simulink model "local_maxima_findpeaks"  (R2019b)
settings: Solver=VariableStepAuto  StartTime=0.0  StopTime=10  RelTol=1e-3
libraries: simulink x2, hdlsllib x1
settings Model: Creator=sbuccelli  LastModifiedBy=sbuccelli

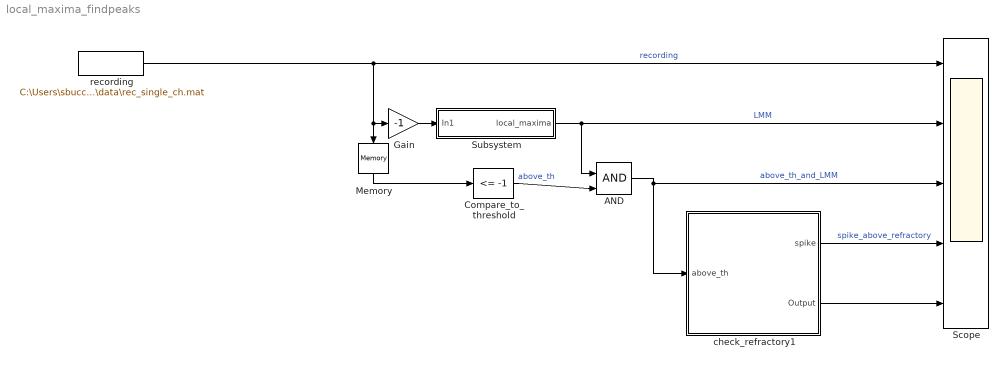
== system local_maxima_findpeaks ==
  AND : Logic  IconShape=distinctive  AllPortsSameDT=off  OutDataTypeStr=boolean
  Compare_to_threshold : simulink/Logic and Bit Operations/Compare To Constant  relop=<=  const=-1  OutDataTypeStr=boolean
  Gain : Gain  Gain=-1
  Memory : Memory  InheritSampleTime=on
  Scope : Scope  NumInputPorts=5
  Subsystem : Subsystem
  check_refractory1 : Subsystem
  recording : FromFile  FileName=C:\Users\sbuccelli\Documents\GitHub\closed-loop-neuroscience\data\rec_single_ch.mat  SampleTime=1/32e3
  wires:
  recording/1 -> Memory/1, Gain/1, Scope/1  "recording"
  AND/1 -> check_refractory1/1(above_th), Scope/3  "above_th_and_LMM"
  check_refractory1/1(spike) -> Scope/4  "spike_above_refractory"
  check_refractory1/2(Output) -> Scope/5
  Subsystem/1(local_maxima) -> AND/1, Scope/2  "LMM"
  Memory/1 -> Compare_to_threshold/1
  Compare_to_threshold/1 -> AND/2  "above_th"
  Gain/1 -> Subsystem/1(In1)

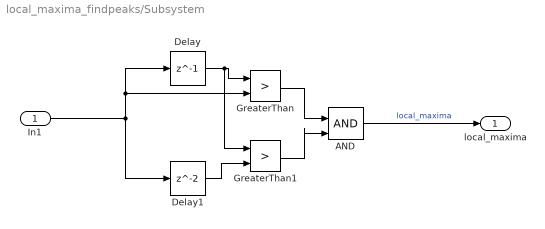
== system local_maxima_findpeaks/Subsystem ==
  In1 : Inport
  AND : Logic  IconShape=distinctive  AllPortsSameDT=off  OutDataTypeStr=boolean
  Delay : Delay  DelayLength=1
  Delay1 : Delay
  GreaterThan : RelationalOperator  Operator=>  OutDataTypeStr=boolean  RndMeth=Simplest
  GreaterThan1 : RelationalOperator  Operator=>  OutDataTypeStr=boolean  RndMeth=Simplest
  local_maxima : Outport
  wires:
  Delay1/1 -> GreaterThan1/2
  GreaterThan1/1 -> AND/2
  GreaterThan/1 -> AND/1
  Delay/1 -> GreaterThan1/1, GreaterThan/1
  AND/1 -> local_maxima/1  "local_maxima"
  In1/1 -> Delay/1, GreaterThan/2, Delay1/1

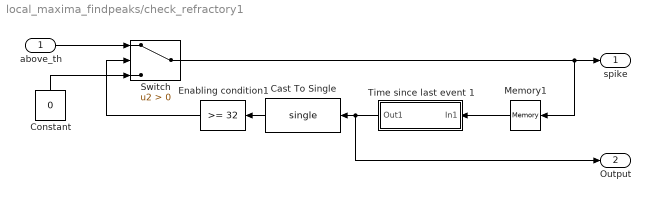
== system local_maxima_findpeaks/check_refractory1 ==
  above_th : Inport
  Cast To Single : DataTypeConversion  OutDataTypeStr=single
  Constant : Constant  Value=0  OutDataTypeStr=boolean
  Enabling condition1 : simulink/Logic and Bit Operations/Compare To Constant  relop=>=  const=32  OutDataTypeStr=boolean
  Memory1 : Memory  InheritSampleTime=on
  Switch : Switch  Criteria=u2 > Threshold
  Time since last event 1 : Subsystem
  spike : Outport
  Output : Outport  Port=2
  wires:
  Switch/1 -> spike/1, Memory1/1
  above_th/1 -> Switch/1
  Memory1/1 -> Time since last event 1/1(In1)
  Time since last event 1/1(Out1) -> Output/1, Cast To Single/1
  Enabling condition1/1 -> Switch/2
  Constant/1 -> Switch/3
  Cast To Single/1 -> Enabling condition1/1

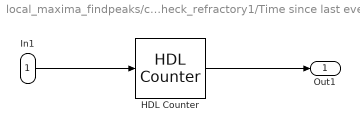
== system local_maxima_findpeaks/check_refractory1/Time since last event 1 ==
  In1 : Inport
  HDL Counter : hdlsllib/Sources/HDL Counter  CountType=Free running  CountInit=1  CountStep=1  CountMax=25  CountFromType=Initial value  CountFrom=1  CountResetPort=on  CountLoadPort=off  CountEnbPort=off  CountDirPort=off  CountDataType=Unsigned  CountWordLen=32  CountFracLen=0  CountSampTime=1
      settings: SourceProductName=Simulink
  Out1 : Outport
  wires:
  In1/1 -> HDL Counter/1
  HDL Counter/1 -> Out1/1
